simulink model "satellite_sim2"  (R2016b)
settings: Solver=ode45  StartTime=0.0  StopTime=10000  RelTol=1e-3  EnableMultiTasking=on
InitFcn:
  | addpath ./..
  | satellite_param
undefined symbols (not defined in the file): P, satellite_animation
settings Model: Creator=beard  LastModifiedBy=beard
settings DataIOCC: LimitDataPoints=on  SaveFormat=Array  SignalLoggingSaveFormat=ModelDataLogs
settings OptimizationCC: ExpressionDepthLimit=2147483647  InitFltsAndDblsToZero=on  LifeSpan=inf
settings DebuggingCC: UnderspecifiedInitializationDetection=Classic  MergeDetectMultiDrivingBlocksExec=none  SolverPrmCheckMsg=warning  FcnCallInpInsideContextMsg=warning  StateNameClashWarn=warning  SFUnexpectedBacktrackingDiag=warning  SFNoUnconditionalDefaultTransitionDiag=warning  SFExecutionAtInitializationDiag=none
settings HardwareCC: ProdBitPerPointer=32  ProdBitPerSizeT=32  ProdBitPerPtrDiffT=32  ProdLargestAtomicFloat=None  ProdIntDivRoundTo=Undefined  ProdEndianess=Unspecified  ProdWordSize=32  ProdHWDeviceType=32-bit Generic
settings ModelReferenceCC: PropagateSignalLabelsOutOfModel=off
settings GRTTargetCC: TargetLangStandard=C89/C90 (ANSI)  GeneratePreprocessorConditionals=Disable all  CombineOutputUpdateFcns=off  GRTInterface=on
settings ConfigComp: CovMetricSettings=dw  CovHtmlReporting=on  CovSaveCumulativeToWorkspaceVar=on  CovSaveSingleToWorkspaceVar=on  CovExternalEMLEnable=off

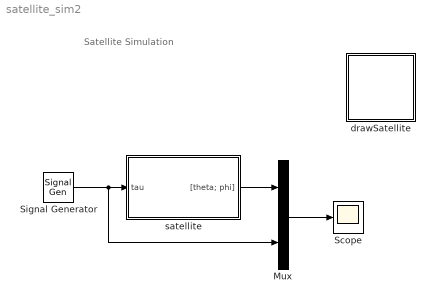
== system satellite_sim2 ==
  note: Satellite Simulation
  Mux : Mux  Inputs=[2;1]
  Scope : Scope
  Signal Generator : SignalGenerator  Frequency=.05
  drawSatellite : Subsystem
      mask Display: image(imread('tv.jpg'))
  satellite : Subsystem
  wires:
  Signal Generator/1 -> Mux/2, satellite/1(tau)
  satellite/1("[theta; phi]") -> Mux/1
  Mux/1 -> Scope/1

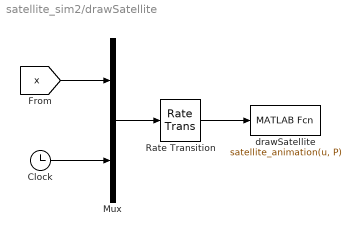
== system satellite_sim2/drawSatellite ==
  Clock : Clock
  Mux : Mux  Inputs=2
  Rate Transition : RateTransition  OutPortSampleTime=P.t_plot
  drawSatellite : MATLABFcn  MATLABFcn=satellite_animation(u, P)  OutputDimensions=0
  wires:
  Mux/1 -> Rate Transition/1
  [x] -> Mux/1
  Clock/1 -> Mux/2
  Rate Transition/1 -> drawSatellite/1

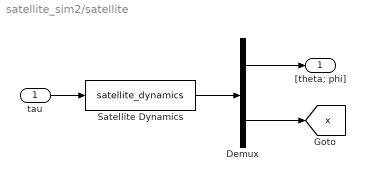
== system satellite_sim2/satellite ==
  tau : Inport
  Demux : Demux  Outputs=[2;4]
  Satellite Dynamics : S-Function  FunctionName=satellite_dynamics  Parameters=P  SFunctionDeploymentMode=off  EnableBusSupport=off
  "[theta; phi]" : Outport
  tag scope: x=global
  wires:
  tau/1 -> Satellite Dynamics/1
  Satellite Dynamics/1 -> Demux/1
  Demux/1 -> "[theta; phi]"/1
  Demux/2 -> [x]
